simulink model "robotarm"  (R2018b)
settings: Solver=FixedStepAuto  StartTime=0.0  StopTime=20  RelTol=1e-3  AbsTol=1e-6
undefined symbols (not defined in the file or in its folder): options
libraries: neural x132, simulink x2
(part 4 of 6)

== system robotarm/NN/Layer 3/Delays 1 ==
  "p{3}" : Inport  PortDimensions=30
      mask Display: e = 0.06;c1 = [120 230 180]/255;c2 = ([120 230 180]+0)/(256+128);c3 = ([120 230 180]+128)/(256+128);patch([0 1 1 0],[0 0 1 1],c1);patch([0 1 1 1-e 1-e 0+e],[0 0 1 1-e 0+e 0+e],c2);patch([0 0 1 1-e 0+e 0+e],[0 1 1 1-e 1-e 0+e],c3);plot([0 1 1 0 0],[0 0 1 1 0]);
  mux : Mux  Inputs=1
      mask Display: e = 0.06;c1 = [120 150 230]/255;c2 = ([120 150 230]+0)/383;c3 = ([120 150 230]+128)/383;patch([0 1 1 0],[0 0 1 1],c1);patch([0 1 1 1-e 1-e 0+e],[0 0 1 1-e 0+e 0+e],c2);patch([0 0 1 1-e 0+e 0+e],[0 1 1 1-e 1-e 0+e],c3);plot([0 1 1 0 0],[0 0 1 1 0]);disp('Mux')
  "pd{3,2}" : Outport
      mask Display: e = 0.06;c1 = [120 230 180]/255;c2 = ([120 230 180]+0)/(256+128);c3 = ([120 230 180]+128)/(256+128);patch([0 1 1 0],[0 0 1 1],c1);patch([0 1 1 1-e 1-e 0+e],[0 0 1 1-e 0+e 0+e],c2);patch([0 0 1 1-e 0+e 0+e],[0 1 1 1-e 1-e 0+e],c3);plot([0 1 1 0 0],[0 0 1 1 0]);
  wires:
  "p{3}"/1 -> mux/1
  mux/1 -> "pd{3,2}"/1

== system robotarm/NN/Layer 3/LW{3,2} ==
  "ad{3,2}" : Inport  PortDimensions=30
      mask Display: e = 0.06;c1 = [120 230 180]/255;c2 = ([120 230 180]+0)/(256+128);c3 = ([120 230 180]+128)/(256+128);patch([0 1 1 0],[0 0 1 1],c1);patch([0 1 1 1-e 1-e 0+e],[0 0 1 1-e 0+e 0+e],c2);patch([0 0 1 1-e 0+e 0+e],[0 1 1 1-e 1-e 0+e],c3);plot([0 1 1 0 0],[0 0 1 1 0]);
  "IW{3,2}(1,:)'" : Constant  Value=[-0.2429257687340068139203452801666571758687496185302734375;0.27084112865980325413062246298068203032016754150390625;0.11171123032023229371123562714274157769978046417236328125;0.1007651682309970431195011997260735370218753814697265625;-0.0277449866479962010956672457950844545848667621612548828125;0.130673395082744392414753065168042667210102081298828125;-0.042123272246463179524500475281456601805984973907470703125;-0.003203601643037117842338634687848752946592867374420166015625;-0.2618888016622322734150429823785088956356048583984375;-0.142572721625630560726705198248964734375476837158203125;-0.0807629847123800537200821736405487172305583953857421875;0.179393701019374185445798275395645759999752044677734375;0.2488682559031003271865500892090494744479656219482421875;-0.279812819743588125920297215998289175331592559814453125;-0.05814160436766295514399160992979886941611766815185546875;0.1510569633210895046371291527975699864327907562255859375;0.45555316936186984744239225619821809232234954833984375;-0.0975242719497680099483005733418394811451435089111328125;-0.0289836703824843978927194854122717515565454959869384765625;-0.0275873688868812465269098055387075874023139476776123046875;-0.1661145100420680364994296951408614404499530792236328125;0.337128175013739317389394045676453970372676849365234375;-0.075506864506494075772735641294275410473346710205078125;0.1376646334660015791317988487207912839949131011962890625;0.047504591453396631528516280695839668624103069305419921875;-0.1029898169805927021780433960884693078696727752685546875;0.141568819340489204794408806264982558786869049072265625;-0.2635181289780434976677270242362283170223236083984375;-0.2147383041130133951579495033001876436173915863037109375;-0.226769009009765099005306865365128032863140106201171875]
      mask Display: e = 0.06;c1 = [120 150 230]/255;c2 = ([120 150 230]+0)/383;c3 = ([120 150 230]+128)/383;patch([0 1 1 0],[0 0 1 1],c1);patch([0 1 1 1-e 1-e 0+e],[0 0 1 1-e 0+e 0+e],c2);patch([0 0 1 1-e 0+e 0+e],[0 1 1 1-e 1-e 0+e],c3);plot([0 1 1 0 0],[0 0 1 1 0]);disp('weights');
  Mux : Mux  Inputs=1
      mask Display: e = 0.06;c1 = [120 150 230]/255;c2 = ([120 150 230]+0)/383;c3 = ([120 150 230]+128)/383;patch([0 1 1 0],[0 0 1 1],c1);patch([0 1 1 1-e 1-e 0+e],[0 0 1 1-e 0+e 0+e],c2);patch([0 0 1 1-e 0+e 0+e],[0 1 1 1-e 1-e 0+e],c3);plot([0 1 1 0 0],[0 0 1 1 0]);disp('Mux');
  dotprod1 : neural/Weight Functions/dotprod
  "lz{3,2}" : Outport
      mask Display: e = 0.06;c1 = [120 230 180]/255;c2 = ([120 230 180]+0)/(256+128);c3 = ([120 230 180]+128)/(256+128);patch([0 1 1 0],[0 0 1 1],c1);patch([0 1 1 1-e 1-e 0+e],[0 0 1 1-e 0+e 0+e],c2);patch([0 0 1 1-e 0+e 0+e],[0 1 1 1-e 1-e 0+e],c3);plot([0 1 1 0 0],[0 0 1 1 0]);
  wires:
  "IW{3,2}(1,:)'"/1 -> dotprod1/1
  "ad{3,2}"/1 -> dotprod1/2
  dotprod1/1 -> Mux/1
  Mux/1 -> "lz{3,2}"/1

== system robotarm/NN_cex_1/Layer 1/Delays 1 ==
  "p{1}" : Inport  PortDimensions=10
      mask Display: e = 0.06;c1 = [120 230 180]/255;c2 = ([120 230 180]+0)/(256+128);c3 = ([120 230 180]+128)/(256+128);patch([0 1 1 0],[0 0 1 1],c1);patch([0 1 1 1-e 1-e 0+e],[0 0 1 1-e 0+e 0+e],c2);patch([0 0 1 1-e 0+e 0+e],[0 1 1 1-e 1-e 0+e],c3);plot([0 1 1 0 0],[0 0 1 1 0]);
  mux : Mux  Inputs=1
      mask Display: e = 0.06;c1 = [120 150 230]/255;c2 = ([120 150 230]+0)/383;c3 = ([120 150 230]+128)/383;patch([0 1 1 0],[0 0 1 1],c1);patch([0 1 1 1-e 1-e 0+e],[0 0 1 1-e 0+e 0+e],c2);patch([0 0 1 1-e 0+e 0+e],[0 1 1 1-e 1-e 0+e],c3);plot([0 1 1 0 0],[0 0 1 1 0]);disp('Mux')
  "pd{1,1}" : Outport
      mask Display: e = 0.06;c1 = [120 230 180]/255;c2 = ([120 230 180]+0)/(256+128);c3 = ([120 230 180]+128)/(256+128);patch([0 1 1 0],[0 0 1 1],c1);patch([0 1 1 1-e 1-e 0+e],[0 0 1 1-e 0+e 0+e],c2);patch([0 0 1 1-e 0+e 0+e],[0 1 1 1-e 1-e 0+e],c3);plot([0 1 1 0 0],[0 0 1 1 0]);
  wires:
  "p{1}"/1 -> mux/1
  mux/1 -> "pd{1,1}"/1

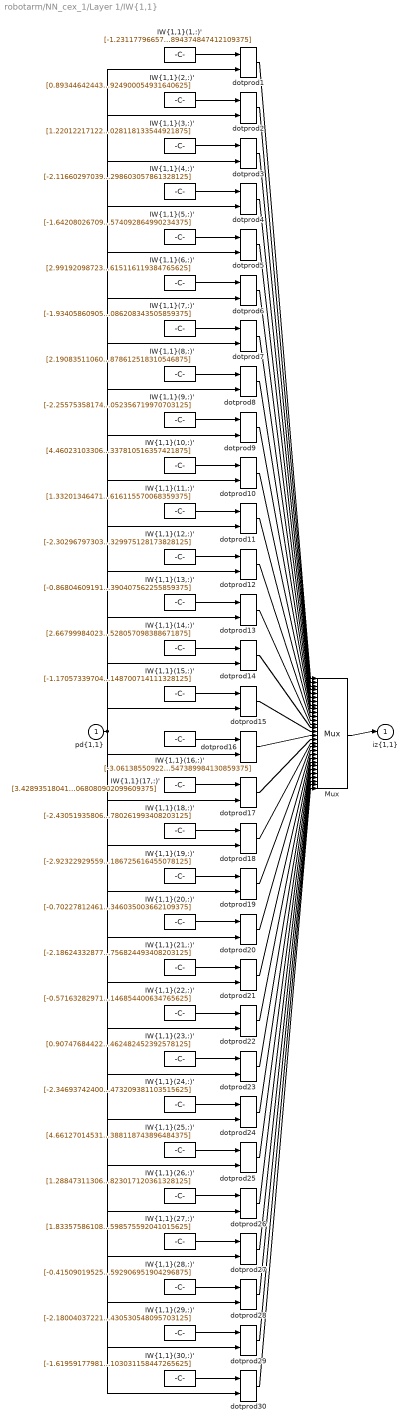
== system robotarm/NN_cex_1/Layer 1/IW{1,1} ==
  "pd{1,1}" : Inport  PortDimensions=10
      mask Display: e = 0.06;c1 = [120 230 180]/255;c2 = ([120 230 180]+0)/(256+128);c3 = ([120 230 180]+128)/(256+128);patch([0 1 1 0],[0 0 1 1],c1);patch([0 1 1 1-e 1-e 0+e],[0 0 1 1-e 0+e 0+e],c2);patch([0 0 1 1-e 0+e 0+e],[0 1 1 1-e 1-e 0+e],c3);plot([0 1 1 0 0],[0 0 1 1 0]);
  "IW{1,1}(1,:)'" : Constant  Value=[-1.2311779665734523536713140856591053307056427001953125;0.83510614378117165035320113020134158432483673095703125;-1.0285958899030152036147001126664690673351287841796875;0.08491753395174884977425477927681640721857547760009765625;0.69300107593370319225556386300013400614261627197265625;-0.35181372632550800272355218112352304160594940185546875;0.5962891267607164369479733068146742880344390869140625;-0.30350245637023276490396028748364187777042388916015625;-0.435084881996784300639546927413903176784515380859375;0.7216321082865382319226910112774930894374847412109375]
      mask Display: e = 0.06;c1 = [120 150 230]/255;c2 = ([120 150 230]+0)/383;c3 = ([120 150 230]+128)/383;patch([0 1 1 0],[0 0 1 1],c1);patch([0 1 1 1-e 1-e 0+e],[0 0 1 1-e 0+e 0+e],c2);patch([0 0 1 1-e 0+e 0+e],[0 1 1 1-e 1-e 0+e],c3);plot([0 1 1 0 0],[0 0 1 1 0]);disp('Weights');
  "IW{1,1}(10,:)'" : Constant  Value=[4.4602310330683412331609360990114510059356689453125;0.1855270466052282019031594018088071607053279876708984375;0.755080240032244720538301407941617071628570556640625;3.020205891292758071386970186722464859485626220703125;-2.0657044909416004685454026912339031696319580078125;-0.55520715910567697282118615476065315306186676025390625;-1.0943877568164694924490731864352710545063018798828125;-0.4203833885407011194956794497556984424591064453125;0.67217171386203899974276509965420700609683990478515625;-1.422385852974535236370456914301030337810516357421875]
      mask Display: e = 0.06;c1 = [120 150 230]/255;c2 = ([120 150 230]+0)/383;c3 = ([120 150 230]+128)/383;patch([0 1 1 0],[0 0 1 1],c1);patch([0 1 1 1-e 1-e 0+e],[0 0 1 1-e 0+e 0+e],c2);patch([0 0 1 1-e 0+e 0+e],[0 1 1 1-e 1-e 0+e],c3);plot([0 1 1 0 0],[0 0 1 1 0]);disp('Weights');
  "IW{1,1}(11,:)'" : Constant  Value=[1.33201346471326242948407525545917451381683349609375;-1.2643459959102327783142527550808154046535491943359375;-1.9317855433305550771905245710513554513454437255859375;0.60593194410617645662142649598536081612110137939453125;0.452475944495226822805733490895363502204418182373046875;0.484921681308493834894335350327310152351856231689453125;1.13070195261233497063813047134317457675933837890625;0.50183487258402792452471885553677566349506378173828125;-0.8321564896213953232972926343791186809539794921875;-2.228002792754578020861799814156256616115570068359375]
      mask Display: e = 0.06;c1 = [120 150 230]/255;c2 = ([120 150 230]+0)/383;c3 = ([120 150 230]+128)/383;patch([0 1 1 0],[0 0 1 1],c1);patch([0 1 1 1-e 1-e 0+e],[0 0 1 1-e 0+e 0+e],c2);patch([0 0 1 1-e 0+e 0+e],[0 1 1 1-e 1-e 0+e],c3);plot([0 1 1 0 0],[0 0 1 1 0]);disp('Weights');
  "IW{1,1}(12,:)'" : Constant  Value=[-2.302967973037755466947373861330561339855194091796875;3.678910338733314855375056140474043786525726318359375;-0.86760414200318758393137841267162002623081207275390625;-0.040295541827813717572492890894864103756844997406005859375;-1.0006627950431397078290274293976835906505584716796875;-0.24134042108036257712200267633306793868541717529296875;-1.0096779553821357833243155255331657826900482177734375;1.337708892780741454231474563130177557468414306640625;0.1757350428759232030540005098373512737452983856201171875;-1.249972727107988124117810002644546329975128173828125]
      mask Display: e = 0.06;c1 = [120 150 230]/255;c2 = ([120 150 230]+0)/383;c3 = ([120 150 230]+128)/383;patch([0 1 1 0],[0 0 1 1],c1);patch([0 1 1 1-e 1-e 0+e],[0 0 1 1-e 0+e 0+e],c2);patch([0 0 1 1-e 0+e 0+e],[0 1 1 1-e 1-e 0+e],c3);plot([0 1 1 0 0],[0 0 1 1 0]);disp('Weights');
  "IW{1,1}(13,:)'" : Constant  Value=[-0.8680460919184185275554455074598081409931182861328125;-0.188443833657483128529719351718085817992687225341796875;0.16776636849725379274644865290611051023006439208984375;-0.010400596202421057145937055565809714607894420623779296875;-0.33063575818592993993405571018229238688945770263671875;0.311320644979175720212793976315879262983798980712890625;-0.2091458705820863628321859550851513631641864776611328125;-1.3844757841136379195035033262684009969234466552734375;-0.2019351548435675824944013356798677705228328704833984375;-0.1495742541834699235181460608146153390407562255859375]
      mask Display: e = 0.06;c1 = [120 150 230]/255;c2 = ([120 150 230]+0)/383;c3 = ([120 150 230]+128)/383;patch([0 1 1 0],[0 0 1 1],c1);patch([0 1 1 1-e 1-e 0+e],[0 0 1 1-e 0+e 0+e],c2);patch([0 0 1 1-e 0+e 0+e],[0 1 1 1-e 1-e 0+e],c3);plot([0 1 1 0 0],[0 0 1 1 0]);disp('Weights');
  "IW{1,1}(14,:)'" : Constant  Value=[2.66799984023553005130224846652708947658538818359375;-2.0562763890653972254085601889528334140777587890625;-0.040382414933480069441085191783713526092469692230224609375;1.0689937110288847410544121885322965681552886962890625;0.3509130364549406522201024927198886871337890625;1.3812072875463010657171025741263292729854583740234375;-1.0773116534716116188263868025387637317180633544921875;-0.2466408501922793539140599250458762980997562408447265625;1.99021030481090033248392501263879239559173583984375;1.4021600102236930762700239938567392528057098388671875]
      mask Display: e = 0.06;c1 = [120 150 230]/255;c2 = ([120 150 230]+0)/383;c3 = ([120 150 230]+128)/383;patch([0 1 1 0],[0 0 1 1],c1);patch([0 1 1 1-e 1-e 0+e],[0 0 1 1-e 0+e 0+e],c2);patch([0 0 1 1-e 0+e 0+e],[0 1 1 1-e 1-e 0+e],c3);plot([0 1 1 0 0],[0 0 1 1 0]);disp('Weights');
  "IW{1,1}(15,:)'" : Constant  Value=[-1.170573397040409080460676705115474760532379150390625;0.384752464233666879867001853199326433241367340087890625;-0.3965715697780682891249171007075347006320953369140625;-1.918703321312856591163154007517732679843902587890625;0.41576794506040204435493023993331007659435272216796875;-0.70684404717127780060081931878812611103057861328125;-0.76185300382311404998603165950044058263301849365234375;-0.14372490518689229332949253148399293422698974609375;1.952000250974990525065777546842582523822784423828125;-1.04612324021826896824904906679876148700714111328125]
      mask Display: e = 0.06;c1 = [120 150 230]/255;c2 = ([120 150 230]+0)/383;c3 = ([120 150 230]+128)/383;patch([0 1 1 0],[0 0 1 1],c1);patch([0 1 1 1-e 1-e 0+e],[0 0 1 1-e 0+e 0+e],c2);patch([0 0 1 1-e 0+e 0+e],[0 1 1 1-e 1-e 0+e],c3);plot([0 1 1 0 0],[0 0 1 1 0]);disp('Weights');
  "IW{1,1}(16,:)'" : Constant  Value=[-3.0613855092209600883279563277028501033782958984375;-0.60346165299476606236339648603461682796478271484375;1.1766197896149594992465381437796168029308319091796875;-1.6419197095252211493487948246183805167675018310546875;0.415118343051256111220226330260629765689373016357421875;0.441761770985573842818183720737579278647899627685546875;1.2739812205330978134298902659793384373188018798828125;0.558101061077895810313975744065828621387481689453125;-0.7226191847052378935956085115321911871433258056640625;1.30848888992569012401645522913895547389984130859375]
      mask Display: e = 0.06;c1 = [120 150 230]/255;c2 = ([120 150 230]+0)/383;c3 = ([120 150 230]+128)/383;patch([0 1 1 0],[0 0 1 1],c1);patch([0 1 1 1-e 1-e 0+e],[0 0 1 1-e 0+e 0+e],c2);patch([0 0 1 1-e 0+e 0+e],[0 1 1 1-e 1-e 0+e],c3);plot([0 1 1 0 0],[0 0 1 1 0]);disp('Weights');
  "IW{1,1}(17,:)'" : Constant  Value=[3.4289351804150296487705418257974088191986083984375;-3.197767235045246625446679900051094591617584228515625;-0.476727044876798788930472028368967585265636444091796875;-0.169964878593053259070444482858874835073947906494140625;-1.0379119479990850383188671912648715078830718994140625;1.325996578455664209883479998097755014896392822265625;0.80538372119936740833878729972639121115207672119140625;0.53599082873951331418282961749355308711528778076171875;-2.77728870804580463271804546820931136608123779296875;-4.4838058541745677842982331640087068080902099609375]
      mask Display: e = 0.06;c1 = [120 150 230]/255;c2 = ([120 150 230]+0)/383;c3 = ([120 150 230]+128)/383;patch([0 1 1 0],[0 0 1 1],c1);patch([0 1 1 1-e 1-e 0+e],[0 0 1 1-e 0+e 0+e],c2);patch([0 0 1 1-e 0+e 0+e],[0 1 1 1-e 1-e 0+e],c3);plot([0 1 1 0 0],[0 0 1 1 0]);disp('Weights');
  "IW{1,1}(18,:)'" : Constant  Value=[-2.430519358064821222598084204946644604206085205078125;0.3272953100676476712038720506825484335422515869140625;0.97458543394296104356300247673061676323413848876953125;0.1165868693579066028842561308920267038047313690185546875;-1.6612494091538561047372013490530662238597869873046875;-3.594078422470215361528289577108807861804962158203125;-4.4725196732284953071712152450345456600189208984375;-0.37217184414544146608960772937280125916004180908203125;5.38811907638532971986933262087404727935791015625;5.13053097486715348196639752131886780261993408203125]
      mask Display: e = 0.06;c1 = [120 150 230]/255;c2 = ([120 150 230]+0)/383;c3 = ([120 150 230]+128)/383;patch([0 1 1 0],[0 0 1 1],c1);patch([0 1 1 1-e 1-e 0+e],[0 0 1 1-e 0+e 0+e],c2);patch([0 0 1 1-e 0+e 0+e],[0 1 1 1-e 1-e 0+e],c3);plot([0 1 1 0 0],[0 0 1 1 0]);disp('Weights');
  "IW{1,1}(19,:)'" : Constant  Value=[-2.923229295595194177082021269598044455051422119140625;1.9893583888356440869671359905623830854892730712890625;-1.4059493712061208459118688551825471222400665283203125;0.83397944345635710572395282724755816161632537841796875;-0.3484142447651681351317165535874664783477783203125;-0.11425450686008790934788947879496845416724681854248046875;-0.30142366792818198195647028114763088524341583251953125;0.026062916188647276827250465203178464435040950775146484375;3.08636500415914127870564698241651058197021484375;3.34885957836597913939158388529904186725616455078125]
      mask Display: e = 0.06;c1 = [120 150 230]/255;c2 = ([120 150 230]+0)/383;c3 = ([120 150 230]+128)/383;patch([0 1 1 0],[0 0 1 1],c1);patch([0 1 1 1-e 1-e 0+e],[0 0 1 1-e 0+e 0+e],c2);patch([0 0 1 1-e 0+e 0+e],[0 1 1 1-e 1-e 0+e],c3);plot([0 1 1 0 0],[0 0 1 1 0]);disp('Weights');
  "IW{1,1}(2,:)'" : Constant  Value=[0.89344642443014976596060705560375936329364776611328125;-0.95836462042056858035010691310162656009197235107421875;0.202076241948744683707417379991966299712657928466796875;-0.495040728966053389381585247974726371467113494873046875;1.542247052320962819038641100632958114147186279296875;-0.272770513253470181513904435632866807281970977783203125;0.1449061285201379833953438946991809643805027008056640625;0.09998208316263991479733164169374504126608371734619140625;1.565989936283480599144013467594049870967864990234375;0.64387085793493670227150005302974022924900054931640625]
      mask Display: e = 0.06;c1 = [120 150 230]/255;c2 = ([120 150 230]+0)/383;c3 = ([120 150 230]+128)/383;patch([0 1 1 0],[0 0 1 1],c1);patch([0 1 1 1-e 1-e 0+e],[0 0 1 1-e 0+e 0+e],c2);patch([0 0 1 1-e 0+e 0+e],[0 1 1 1-e 1-e 0+e],c3);plot([0 1 1 0 0],[0 0 1 1 0]);disp('Weights');
  "IW{1,1}(20,:)'" : Constant  Value=[-0.70227812461453920089837765772244893014430999755859375;1.5184923834467765058064969707629643380641937255859375;0.43995337665290390471994896870455704629421234130859375;0.948058535887257303187425350188277661800384521484375;0.11783968768984835751023609873300301842391490936279296875;-0.50048984438261145957227427061297930777072906494140625;0.267089119537599228859647837452939711511135101318359375;0.277483938140590857823752912736381404101848602294921875;-0.94420115262839232617153584214975126087665557861328125;0.76594241653026207128363012088811956346035003662109375]
      mask Display: e = 0.06;c1 = [120 150 230]/255;c2 = ([120 150 230]+0)/383;c3 = ([120 150 230]+128)/383;patch([0 1 1 0],[0 0 1 1],c1);patch([0 1 1 1-e 1-e 0+e],[0 0 1 1-e 0+e 0+e],c2);patch([0 0 1 1-e 0+e 0+e],[0 1 1 1-e 1-e 0+e],c3);plot([0 1 1 0 0],[0 0 1 1 0]);disp('Weights');
  "IW{1,1}(21,:)'" : Constant  Value=[-2.186243328777522254569021242787130177021026611328125;1.8646760496676277885086392416269518435001373291015625;1.1887222203316554214325151406228542327880859375;0.2891522798865826526792943695909343659877777099609375;1.0576561743181980279615572726470418274402618408203125;0.38202195037432973290236759567051194608211517333984375;0.51051231074171876667122660364839248359203338623046875;0.2064512653605895253772217756704776547849178314208984375;-0.8597415636233385338726975533063523471355438232421875;-1.2913760043427953139172359442454762756824493408203125]
      mask Display: e = 0.06;c1 = [120 150 230]/255;c2 = ([120 150 230]+0)/383;c3 = ([120 150 230]+128)/383;patch([0 1 1 0],[0 0 1 1],c1);patch([0 1 1 1-e 1-e 0+e],[0 0 1 1-e 0+e 0+e],c2);patch([0 0 1 1-e 0+e 0+e],[0 1 1 1-e 1-e 0+e],c3);plot([0 1 1 0 0],[0 0 1 1 0]);disp('Weights');
  "IW{1,1}(22,:)'" : Constant  Value=[-0.57163282971566664603102481123642064630985260009765625;0.2434333217343922217690277420842903666198253631591796875;-0.69726556097993797056489029273507185280323028564453125;1.912292585860537297293149094912223517894744873046875;-1.087795208161920879064155087689869105815887451171875;1.036359990688623611276852898299694061279296875;0.214953565502753296545535022232797928154468536376953125;0.188551761370062853639950617434806190431118011474609375;0.88967459126058312524065740944934077560901641845703125;-0.83026710294146843782669975553289987146854400634765625]
      mask Display: e = 0.06;c1 = [120 150 230]/255;c2 = ([120 150 230]+0)/383;c3 = ([120 150 230]+128)/383;patch([0 1 1 0],[0 0 1 1],c1);patch([0 1 1 1-e 1-e 0+e],[0 0 1 1-e 0+e 0+e],c2);patch([0 0 1 1-e 0+e 0+e],[0 1 1 1-e 1-e 0+e],c3);plot([0 1 1 0 0],[0 0 1 1 0]);disp('Weights');
  "IW{1,1}(23,:)'" : Constant  Value=[0.9074768442268228429981036242679692804813385009765625;-0.560640227443274685725782546796835958957672119140625;0.213378386503975281396350283102947287261486053466796875;0.026170108031081627808500655874013318680226802825927734375;-0.72017074879963782763070412329398095607757568359375;-1.24645810289776459711674760910682380199432373046875;-1.098738136930617059761061682365834712982177734375;-1.016317926270413618539123490336351096630096435546875;-0.90018551544646430162543992992141284048557281494140625;0.053341516463971949679745421235566027462482452392578125]
      mask Display: e = 0.06;c1 = [120 150 230]/255;c2 = ([120 150 230]+0)/383;c3 = ([120 150 230]+128)/383;patch([0 1 1 0],[0 0 1 1],c1);patch([0 1 1 1-e 1-e 0+e],[0 0 1 1-e 0+e 0+e],c2);patch([0 0 1 1-e 0+e 0+e],[0 1 1 1-e 1-e 0+e],c3);plot([0 1 1 0 0],[0 0 1 1 0]);disp('Weights');
  "IW{1,1}(24,:)'" : Constant  Value=[-2.346937424003892491697342848055996000766754150390625;1.966051328208128889940553563064895570278167724609375;0.874848814916065808944267701008357107639312744140625;0.356823534058804792135077832426759414374828338623046875;0.77439141593680138608846164061105810105800628662109375;-0.402606514271772741864197087124921381473541259765625;-0.71878958941472437249586846519378013908863067626953125;0.73358206461505248707766213556169532239437103271484375;2.657186630809629246385838996502570807933807373046875;1.6036623859711041095721384408534504473209381103515625]
      mask Display: e = 0.06;c1 = [120 150 230]/255;c2 = ([120 150 230]+0)/383;c3 = ([120 150 230]+128)/383;patch([0 1 1 0],[0 0 1 1],c1);patch([0 1 1 1-e 1-e 0+e],[0 0 1 1-e 0+e 0+e],c2);patch([0 0 1 1-e 0+e 0+e],[0 1 1 1-e 1-e 0+e],c3);plot([0 1 1 0 0],[0 0 1 1 0]);disp('Weights');
  "IW{1,1}(25,:)'" : Constant  Value=[4.66127014531470962310777395032346248626708984375;-3.52772594621653379221015711664222180843353271484375;-0.71021563618010297158633647995884530246257781982421875;0.95331774478694442098714034727890975773334503173828125;-1.1660178684885462718767712431144900619983673095703125;-0.86562658481946763711079029235406778752803802490234375;-0.5928704844969374665453187844832427799701690673828125;-0.1280771288915418526510592300837743096053600311279296875;-1.226155349971019159482921168091706931591033935546875;-1.28403667011046618284808573662303388118743896484375]
      mask Display: e = 0.06;c1 = [120 150 230]/255;c2 = ([120 150 230]+0)/383;c3 = ([120 150 230]+128)/383;patch([0 1 1 0],[0 0 1 1],c1);patch([0 1 1 1-e 1-e 0+e],[0 0 1 1-e 0+e 0+e],c2);patch([0 0 1 1-e 0+e 0+e],[0 1 1 1-e 1-e 0+e],c3);plot([0 1 1 0 0],[0 0 1 1 0]);disp('Weights');
  "IW{1,1}(26,:)'" : Constant  Value=[1.28847311306085199333892887807451188564300537109375;-1.6797808592658280968379358455422334372997283935546875;-2.144618861386469621521655426477082073688507080078125;1.0097300090442271613966340737533755600452423095703125;-2.027854394738220822347329885815270245075225830078125;-0.927126679965457167753584144520573318004608154296875;-1.8842765269497210312010793131776154041290283203125;0.484327072961073967771739035015343688428401947021484375;2.2063049245424206645793674397282302379608154296875;2.25787943841652793963703516055829823017120361328125]
      mask Display: e = 0.06;c1 = [120 150 230]/255;c2 = ([120 150 230]+0)/383;c3 = ([120 150 230]+128)/383;patch([0 1 1 0],[0 0 1 1],c1);patch([0 1 1 1-e 1-e 0+e],[0 0 1 1-e 0+e 0+e],c2);patch([0 0 1 1-e 0+e 0+e],[0 1 1 1-e 1-e 0+e],c3);plot([0 1 1 0 0],[0 0 1 1 0]);disp('Weights');
  "IW{1,1}(27,:)'" : Constant  Value=[1.8335758610809731461444016531459055840969085693359375;-0.80033649236045334429690001343260519206523895263671875;0.62995976636199546572214558182167820632457733154296875;-0.310666019422124073390278908846084959805011749267578125;1.0664849117267867217861976314452476799488067626953125;-0.8488324072187409807810354323009960353374481201171875;-0.1266700969891333683481349225985468365252017974853515625;-0.70971618693911475705959901461028493940830230712890625;-1.61942996775658176744627780863083899021148681640625;-1.838435776806305543829012094647623598575592041015625]
      mask Display: e = 0.06;c1 = [120 150 230]/255;c2 = ([120 150 230]+0)/383;c3 = ([120 150 230]+128)/383;patch([0 1 1 0],[0 0 1 1],c1);patch([0 1 1 1-e 1-e 0+e],[0 0 1 1-e 0+e 0+e],c2);patch([0 0 1 1-e 0+e 0+e],[0 1 1 1-e 1-e 0+e],c3);plot([0 1 1 0 0],[0 0 1 1 0]);disp('Weights');
  "IW{1,1}(28,:)'" : Constant  Value=[-0.415090195251639482165728622931055724620819091796875;2.31131568197506798156837248825468122959136962890625;2.46872726633397832074479083530604839324951171875;1.4915796824353495519943635372328571975231170654296875;0.380927243432112760945784657451440580189228057861328125;0.6753681782011577983126926483237184584140777587890625;-0.54177915469498205691678549555945210158824920654296875;0.8365811769897562033548865656484849750995635986328125;-0.5148571282281146910264624239061959087848663330078125;0.3409485684322877130369988663005642592906951904296875]
      mask Display: e = 0.06;c1 = [120 150 230]/255;c2 = ([120 150 230]+0)/383;c3 = ([120 150 230]+128)/383;patch([0 1 1 0],[0 0 1 1],c1);patch([0 1 1 1-e 1-e 0+e],[0 0 1 1-e 0+e 0+e],c2);patch([0 0 1 1-e 0+e 0+e],[0 1 1 1-e 1-e 0+e],c3);plot([0 1 1 0 0],[0 0 1 1 0]);disp('Weights');
  "IW{1,1}(29,:)'" : Constant  Value=[-2.18004037221372559685050873667933046817779541015625;2.57953362757347992584300300222821533679962158203125;0.14238786549321924557176544112735427916049957275390625;0.55241863538390545418366173180402256548404693603515625;-0.4687675311390100407749059741036035120487213134765625;1.111195383273993808614932277123443782329559326171875;-1.816992848019115314173177466727793216705322265625;0.08084522952570878662204023612503078766167163848876953125;1.3506280386167037743661012427764944732189178466796875;2.59044112871999487879293155856430530548095703125]
      mask Display: e = 0.06;c1 = [120 150 230]/255;c2 = ([120 150 230]+0)/383;c3 = ([120 150 230]+128)/383;patch([0 1 1 0],[0 0 1 1],c1);patch([0 1 1 1-e 1-e 0+e],[0 0 1 1-e 0+e 0+e],c2);patch([0 0 1 1-e 0+e 0+e],[0 1 1 1-e 1-e 0+e],c3);plot([0 1 1 0 0],[0 0 1 1 0]);disp('Weights');
  "IW{1,1}(3,:)'" : Constant  Value=[1.220122171225292984075849744840525090694427490234375;0.268762870353162430792082204789039678871631622314453125;-1.37905066247729291006862695212475955486297607421875;1.215024517010909743675028948928229510784149169921875;-1.693434820109444682856292274664156138896942138671875;0.5272954595371450725593831521109677851200103759765625;0.0261466447854443208298480527673746109940111637115478515625;-0.34655282192955805253831158552202396094799041748046875;-0.062423356704078357404252841433844878338277339935302734375;-1.7795392593944832082542006901348941028118133544921875]
      mask Display: e = 0.06;c1 = [120 150 230]/255;c2 = ([120 150 230]+0)/383;c3 = ([120 150 230]+128)/383;patch([0 1 1 0],[0 0 1 1],c1);patch([0 1 1 1-e 1-e 0+e],[0 0 1 1-e 0+e 0+e],c2);patch([0 0 1 1-e 0+e 0+e],[0 1 1 1-e 1-e 0+e],c3);plot([0 1 1 0 0],[0 0 1 1 0]);disp('Weights');
  "IW{1,1}(30,:)'" : Constant  Value=[-1.6195917798102310580787843719008378684520721435546875;2.868136096518615563155663039651699364185333251953125;-0.148988772405738545412390294586657546460628509521484375;-0.269127305674739136787110282966750673949718475341796875;1.1026460308094805373713143126224167644977569580078125;0.60721268475408340936638751372811384499073028564453125;-0.69552233010687014580497589122387580573558807373046875;1.1339742309767959493882472088444046676158905029296875;0.1633210715633823806314239845960400998592376708984375;-0.1317878662916322218823239609264419414103031158447265625]
      mask Display: e = 0.06;c1 = [120 150 230]/255;c2 = ([120 150 230]+0)/383;c3 = ([120 150 230]+128)/383;patch([0 1 1 0],[0 0 1 1],c1);patch([0 1 1 1-e 1-e 0+e],[0 0 1 1-e 0+e 0+e],c2);patch([0 0 1 1-e 0+e 0+e],[0 1 1 1-e 1-e 0+e],c3);plot([0 1 1 0 0],[0 0 1 1 0]);disp('Weights');
  "IW{1,1}(4,:)'" : Constant  Value=[-2.116602970397174043881705074454657733440399169921875;2.0542617615480782689019179088063538074493408203125;-0.38152233474946317670628559426404535770416259765625;1.987920703461345084406275418587028980255126953125;0.5431003151797728634164741379208862781524658203125;-0.75789726692708281330368436101707629859447479248046875;-0.2343991331290598834069527356405160389840602874755859375;0.50243058964974240954148854143568314611911773681640625;-0.75292730502721927354770059537258930504322052001953125;0.492710948674372872790883093330194242298603057861328125]
      mask Display: e = 0.06;c1 = [120 150 230]/255;c2 = ([120 150 230]+0)/383;c3 = ([120 150 230]+128)/383;patch([0 1 1 0],[0 0 1 1],c1);patch([0 1 1 1-e 1-e 0+e],[0 0 1 1-e 0+e 0+e],c2);patch([0 0 1 1-e 0+e 0+e],[0 1 1 1-e 1-e 0+e],c3);plot([0 1 1 0 0],[0 0 1 1 0]);disp('Weights');
  "IW{1,1}(5,:)'" : Constant  Value=[-1.64208026709051768676772553590126335620880126953125;-0.234870704537322172456015323405154049396514892578125;1.1271578460713131963899513721116818487644195556640625;-0.9834519611389531679179754064534790813922882080078125;-0.73568627300666589174937826101086102426052093505859375;0.1256510048179040606175504990460467524826526641845703125;0.8123861716682991840343674994073808193206787109375;1.5532338304348101143403937385301105678081512451171875;-1.250776568059308591074341165949590504169464111328125;0.065537127640976799991534562650485895574092864990234375]
      mask Display: e = 0.06;c1 = [120 150 230]/255;c2 = ([120 150 230]+0)/383;c3 = ([120 150 230]+128)/383;patch([0 1 1 0],[0 0 1 1],c1);patch([0 1 1 1-e 1-e 0+e],[0 0 1 1-e 0+e 0+e],c2);patch([0 0 1 1-e 0+e 0+e],[0 1 1 1-e 1-e 0+e],c3);plot([0 1 1 0 0],[0 0 1 1 0]);disp('Weights');
  "IW{1,1}(6,:)'" : Constant  Value=[2.991920987233985140818504078197292983531951904296875;-1.1412705566270695545227908951346762478351593017578125;0.810526656428611769200642811483703553676605224609375;0.853362666216746834635387131129391491413116455078125;-0.253237470513439977271019643012550659477710723876953125;0.59860663936890745606689279156853444874286651611328125;-0.73591047668771059075965013107634149491786956787109375;0.74916212973047269230164602049626410007476806640625;-0.18372172743006787154484982238500379025936126708984375;-0.13636534911503039868563291747705079615116119384765625]
      mask Display: e = 0.06;c1 = [120 150 230]/255;c2 = ([120 150 230]+0)/383;c3 = ([120 150 230]+128)/383;patch([0 1 1 0],[0 0 1 1],c1);patch([0 1 1 1-e 1-e 0+e],[0 0 1 1-e 0+e 0+e],c2);patch([0 0 1 1-e 0+e 0+e],[0 1 1 1-e 1-e 0+e],c3);plot([0 1 1 0 0],[0 0 1 1 0]);disp('Weights');
  "IW{1,1}(7,:)'" : Constant  Value=[-1.934058609055788746644566344912163913249969482421875;1.830275610788592022259990699240006506443023681640625;1.3362432989885373313398986283573321998119354248046875;0.6221061728166972226716779914568178355693817138671875;-1.6988279187389456748036309363669715821743011474609375;0.9057307313014673066930981804034672677516937255859375;-0.3637590704727522439299036705051548779010772705078125;1.119483929420443057978218348580412566661834716796875;1.4774087730884828406630049357772804796695709228515625;-0.36681482805728859997174140517017804086208343505859375]
      mask Display: e = 0.06;c1 = [120 150 230]/255;c2 = ([120 150 230]+0)/383;c3 = ([120 150 230]+128)/383;patch([0 1 1 0],[0 0 1 1],c1);patch([0 1 1 1-e 1-e 0+e],[0 0 1 1-e 0+e 0+e],c2);patch([0 0 1 1-e 0+e 0+e],[0 1 1 1-e 1-e 0+e],c3);plot([0 1 1 0 0],[0 0 1 1 0]);disp('Weights');
  "IW{1,1}(8,:)'" : Constant  Value=[2.190835110600959811932852971949614584445953369140625;-2.717892240790882762979663311853073537349700927734375;-0.570712592603343171759888718952424824237823486328125;0.01174094197304350987998144972834779764525592327117919921875;0.262798479866374334878997842679382301867008209228515625;-0.3312435366636428124564872632618062198162078857421875;0.516534323820891483336481542210094630718231201171875;-0.061294993989314490445696748111004126258194446563720703125;-0.397286796422957666496955653201439417898654937744140625;-0.49527933795716971854261601038160733878612518310546875]
      mask Display: e = 0.06;c1 = [120 150 230]/255;c2 = ([120 150 230]+0)/383;c3 = ([120 150 230]+128)/383;patch([0 1 1 0],[0 0 1 1],c1);patch([0 1 1 1-e 1-e 0+e],[0 0 1 1-e 0+e 0+e],c2);patch([0 0 1 1-e 0+e 0+e],[0 1 1 1-e 1-e 0+e],c3);plot([0 1 1 0 0],[0 0 1 1 0]);disp('Weights');
  "IW{1,1}(9,:)'" : Constant  Value=[-2.255753581740514324138757729087956249713897705078125;0.491138153844949465476332761681987904012203216552734375;-1.8538218472849028461979514759150333702564239501953125;-0.82207084680782127605880305054597556591033935546875;0.250956832680597596851868047451716847717761993408203125;0.034276763484118510927345369054819457232952117919921875;-0.985685100148604664838103417423553764820098876953125;-0.383759935283498332392326801709714345633983612060546875;0.90265763491978978638741182294324971735477447509765625;-0.176278926110774503133171720037353225052356719970703125]
      mask Display: e = 0.06;c1 = [120 150 230]/255;c2 = ([120 150 230]+0)/383;c3 = ([120 150 230]+128)/383;patch([0 1 1 0],[0 0 1 1],c1);patch([0 1 1 1-e 1-e 0+e],[0 0 1 1-e 0+e 0+e],c2);patch([0 0 1 1-e 0+e 0+e],[0 1 1 1-e 1-e 0+e],c3);plot([0 1 1 0 0],[0 0 1 1 0]);disp('Weights');
  Mux : Mux  Inputs=30
      mask Display: e = 0.06;c1 = [120 150 230]/255;c2 = ([120 150 230]+0)/383;c3 = ([120 150 230]+128)/383;patch([0 1 1 0],[0 0 1 1],c1);patch([0 1 1 1-e 1-e 0+e],[0 0 1 1-e 0+e 0+e],c2);patch([0 0 1 1-e 0+e 0+e],[0 1 1 1-e 1-e 0+e],c3);plot([0 1 1 0 0],[0 0 1 1 0]);disp('Mux');
  dotprod{1..30} (30 alike) : neural/Weight Functions/dotprod
  "iz{1,1}" : Outport
      mask Display: e = 0.06;c1 = [120 230 180]/255;c2 = ([120 230 180]+0)/(256+128);c3 = ([120 230 180]+128)/(256+128);patch([0 1 1 0],[0 0 1 1],c1);patch([0 1 1 1-e 1-e 0+e],[0 0 1 1-e 0+e 0+e],c2);patch([0 0 1 1-e 0+e 0+e],[0 1 1 1-e 1-e 0+e],c3);plot([0 1 1 0 0],[0 0 1 1 0]);
  wires:
  "IW{1,1}(1,:)'"/1 -> dotprod1/1
  "pd{1,1}"/1 -> dotprod1/2, dotprod2/2, dotprod3/2, dotprod4/2, dotprod5/2, dotprod6/2, dotprod7/2, dotprod8/2, dotprod9/2, dotprod10/2, dotprod11/2, dotprod12/2, dotprod13/2, dotprod14/2, dotprod15/2, dotprod16/2, dotprod17/2, dotprod18/2, dotprod19/2, dotprod20/2, dotprod21/2, dotprod22/2, dotprod23/2, dotprod24/2, dotprod25/2, dotprod26/2, dotprod27/2, dotprod28/2, dotprod29/2, dotprod30/2
  dotprod1/1 -> Mux/1
  "IW{1,1}(2,:)'"/1 -> dotprod2/1
  dotprod2/1 -> Mux/2
  "IW{1,1}(3,:)'"/1 -> dotprod3/1
  dotprod3/1 -> Mux/3
  "IW{1,1}(4,:)'"/1 -> dotprod4/1
  dotprod4/1 -> Mux/4
  "IW{1,1}(5,:)'"/1 -> dotprod5/1
  dotprod5/1 -> Mux/5
  "IW{1,1}(6,:)'"/1 -> dotprod6/1
  dotprod6/1 -> Mux/6
  "IW{1,1}(7,:)'"/1 -> dotprod7/1
  dotprod7/1 -> Mux/7
  "IW{1,1}(8,:)'"/1 -> dotprod8/1
  dotprod8/1 -> Mux/8
  "IW{1,1}(9,:)'"/1 -> dotprod9/1
  dotprod9/1 -> Mux/9
  "IW{1,1}(10,:)'"/1 -> dotprod10/1
  dotprod10/1 -> Mux/10
  "IW{1,1}(11,:)'"/1 -> dotprod11/1
  dotprod11/1 -> Mux/11
  "IW{1,1}(12,:)'"/1 -> dotprod12/1
  dotprod12/1 -> Mux/12
  "IW{1,1}(13,:)'"/1 -> dotprod13/1
  dotprod13/1 -> Mux/13
  "IW{1,1}(14,:)'"/1 -> dotprod14/1
  dotprod14/1 -> Mux/14
  "IW{1,1}(15,:)'"/1 -> dotprod15/1
  dotprod15/1 -> Mux/15
  "IW{1,1}(16,:)'"/1 -> dotprod16/1
  dotprod16/1 -> Mux/16
  "IW{1,1}(17,:)'"/1 -> dotprod17/1
  dotprod17/1 -> Mux/17
  "IW{1,1}(18,:)'"/1 -> dotprod18/1
  dotprod18/1 -> Mux/18
  "IW{1,1}(19,:)'"/1 -> dotprod19/1
  dotprod19/1 -> Mux/19
  "IW{1,1}(20,:)'"/1 -> dotprod20/1
  dotprod20/1 -> Mux/20
  "IW{1,1}(21,:)'"/1 -> dotprod21/1
  dotprod21/1 -> Mux/21
  "IW{1,1}(22,:)'"/1 -> dotprod22/1
  dotprod22/1 -> Mux/22
  "IW{1,1}(23,:)'"/1 -> dotprod23/1
  dotprod23/1 -> Mux/23
  "IW{1,1}(24,:)'"/1 -> dotprod24/1
  dotprod24/1 -> Mux/24
  "IW{1,1}(25,:)'"/1 -> dotprod25/1
  dotprod25/1 -> Mux/25
  "IW{1,1}(26,:)'"/1 -> dotprod26/1
  dotprod26/1 -> Mux/26
  "IW{1,1}(27,:)'"/1 -> dotprod27/1
  dotprod27/1 -> Mux/27
  "IW{1,1}(28,:)'"/1 -> dotprod28/1
  dotprod28/1 -> Mux/28
  "IW{1,1}(29,:)'"/1 -> dotprod29/1
  dotprod29/1 -> Mux/29
  "IW{1,1}(30,:)'"/1 -> dotprod30/1
  dotprod30/1 -> Mux/30
  Mux/1 -> "iz{1,1}"/1

== system robotarm/NN_cex_1/Layer 2/Delays 1 ==
  "p{2}" : Inport  PortDimensions=30
      mask Display: e = 0.06;c1 = [120 230 180]/255;c2 = ([120 230 180]+0)/(256+128);c3 = ([120 230 180]+128)/(256+128);patch([0 1 1 0],[0 0 1 1],c1);patch([0 1 1 1-e 1-e 0+e],[0 0 1 1-e 0+e 0+e],c2);patch([0 0 1 1-e 0+e 0+e],[0 1 1 1-e 1-e 0+e],c3);plot([0 1 1 0 0],[0 0 1 1 0]);
  mux : Mux  Inputs=1
      mask Display: e = 0.06;c1 = [120 150 230]/255;c2 = ([120 150 230]+0)/383;c3 = ([120 150 230]+128)/383;patch([0 1 1 0],[0 0 1 1],c1);patch([0 1 1 1-e 1-e 0+e],[0 0 1 1-e 0+e 0+e],c2);patch([0 0 1 1-e 0+e 0+e],[0 1 1 1-e 1-e 0+e],c3);plot([0 1 1 0 0],[0 0 1 1 0]);disp('Mux')
  "pd{2,1}" : Outport
      mask Display: e = 0.06;c1 = [120 230 180]/255;c2 = ([120 230 180]+0)/(256+128);c3 = ([120 230 180]+128)/(256+128);patch([0 1 1 0],[0 0 1 1],c1);patch([0 1 1 1-e 1-e 0+e],[0 0 1 1-e 0+e 0+e],c2);patch([0 0 1 1-e 0+e 0+e],[0 1 1 1-e 1-e 0+e],c3);plot([0 1 1 0 0],[0 0 1 1 0]);
  wires:
  "p{2}"/1 -> mux/1
  mux/1 -> "pd{2,1}"/1
